simulink model "AUAV_V3_TestSensors"  (R2015a)
settings: Solver=FixedStepDiscrete  StartTime=0.0  StopTime=10.0  FixedStep=T  RelTol=1e-3
PreLoadFcn:
  | %T = 0.0025;
  | MavlinkBus;
  | mcuInit;
  | % Baro Altitude Computation
  | % =========================
  | basePressure = 98192.64;
  | baseTemp = 288.215;
  | lapseRate = -0.00198122;
  | baseHeight = 0;
values from neighbouring files (symbols this model uses):
  apSampleTime = 0.01    [mcuInit.m]
  latlong_WP = 1    [mcuInit.m]
  mavlink_attitude_t = Simulink.Bus    [MavlinkBusMarcello.m]
  mavlink_gps_raw_int_t = Simulink.Bus    [MavlinkBus.m]    (also in MavlinkBusMarcello.m)
  mavlink_raw_imu_t = Simulink.Bus    [MavlinkBus.m]    (also in MavlinkBusMarcello.m)
  mavlink_scaled_pressure_t = Simulink.Bus    [MavlinkBus.m]    (also in MavlinkBusMarcello.m)
  mavlink_servo_output_raw_t = Simulink.Bus    [MavlinkBusMarcello.m]
  mavlink_slugs_navigation_t = Simulink.Bus    [MavlinkBusMarcello.m]
  mavlink_sys_status_t = Simulink.Bus    [MavlinkBus.m]    (also in MavlinkBusMarcello.m)
  T = 0.01    [mcuInit.m]
  Xpoints = [0 0]    [mcuInit.m]
  Ypoints = [0 0]    [mcuInit.m]
  Zpoints = [0 0]    [mcuInit.m]
undefined symbols (not defined in the file or in its folder): A0, A14, A15, A2, A3, A4, A5, A6, accBiasRateLimit, B0, bankCommandLimit, barAdjust, baroCutoff, baroCutTemp, cubeAccelGain16405, cubeGyroGain16405, cubeMagGain16405, D0, D11, D7, D8, daLimit, data, daTrimMax, daTrimMin, deLimit, deTrimMax, deTrimMin, drLimit, drTrimMax, drTrimMin, dtLimit, dtTrimMax, dtTrimMin, F2, F3, G0, G13, G15, gaind, GS_location, gyroBiasRateLimit, IC1max, IPStar, ISA_g, Max, maxAcc, MaxDwnPthStar, maxDynPressure, maxEta, mlParamInterface, ms, OC1max, P112, P125, P127, P16, P20, P21, P30 ... (+26)
undefined symbols (not defined in the file): baroOffset, baroScale, barTGain1, barTGain2, barTMean1, barTMean2, bda, bde, bdr, bdt, bICda, bICde, bICdr, bICdt, derivativesConstant, lowRateSensorCutoff, mainSensorCutoff, mda, mde, mdr, mdt, mICda, mICde, mICdr, mICdt, pitotOffset, pitotScale, pitTGain1, pitTGain2, pitTMean1, pitTMean2, powerOffset, powerScale, pressureSensorCutoff, tempOffset, tempScale, vzCutoff, xCutoff, yCutoff
libraries: MCHP_Blockset x158, simulink x84, SLUGS_Library x31, aerolibconvert2 x6, aerolibutil x4, aerolibtransform2 x3, dspmtrx3 x2, aerolibobsolete x2
(part 2 of 24)

== system AUAV_V3_TestSensors/Barometer_Driver ==
  In1 : Inport
  BMP 180 Temperature Compensation See datasheet : Subsystem
  "BUS I2C Initialize BMP180 Read P, Convert T° @100Hz" : MCHP_Blockset/BUS I2C/BUS I2C MASTER  I2CRef=2  I2C_IntPriority=6  I2Csequence_txt="Initial-Configuration$     ---     $Start$Write Address:{[0x77]}    % BMP180 Address$Write Data (x1)  Write:{[0xF6]}  $Re-Start    % Re-Start when not followed with either Read or Write action rethrow Address$Read Data (x2)  Read:{adc out}    % Read converted value$Stop$Start$Write Address:{[0x77]}    % BMP180 Address$Write Data (x1)  Write:{[0xF4 0x2E]}      % Start T° Conversion$Stop"  I2Csequence_num=[BFF0000000000000 40E0600000000000 40F86A0000000000 410065D9C7810E65]$[4070000000000000]$[3FF0000000000000 40E0200000000000 40F86A0000000000 40F866E066594CA2]$[4040000000000000 0000000000000000 0000000000000000 405DC00000000000]$[4050000000000000 3FF0000000000000 0000000000000000 406EC00000000000]$[4008000000000000 40E0000000000000 40F86A0000000000 410065D9C7810E65]$[4060000000000000 4000000000000000]$[4000000000000000 40E0000000000000 40F86A0000000000 410065D9C7810E65]$[3FF0000000000000 40E0000000000000 40F86A0000000000 410065D9C7810E65]$[4040000000000000 0000000000000000 0000000000000000 405DC00000000000]$[4050000000000000 3FF0000000000000 0000000000000000 406E800000000000 4047000000000000]$[4000000000000000 40E0000000000000 40F86A0000000000 410065D9C7810E65]  InitialConfigurationNum=0  PIN_SDA_TXT=A3 / Pin[59]  PIN_SCL_TXT=A2 / Pin[58]  S_INPUT="[5  5]"  S_OUTPUT=[5]  S_INPUT_Size="[2  2]"  S_OUTPUT_Size=[4]  BlockingMode=off  SampleTime=[.01]  MCHP_MASTERLINK=|  MCHP_PORT={I2C 2 Clock}{SCL2}13:0:A2;{I2C 2 SDA}{SDA2}13:0:A3;  ORDERING=0
      | AUAV_V3_TestSensors/Microchip Master
      | AUAV V3 Board
      | Busy Flag on D2 (RA6)
  "BUS I2C Initialize BMP180 Read T°, Convert P @ 100Hz" : MCHP_Blockset/BUS I2C/BUS I2C MASTER  I2CRef=2  I2C_IntPriority=6  I2Csequence_txt="Initial-Configuration$     ---     $Start$Write Address:{[0x77]}    % BMP180 Address$Write Data (x1)  Write:{[0xF6]}  $Re-Start    % Re-Start when not followed with either Read or Write action rethrow Address$Read Data (x2)  Read:{adc out}    % Read converted value$Stop$Start$Write Address:{[0x77]}    % BMP180 Address$Write Data (x1)  Write:{[0xF4 0x34]}      % Start T° Conversion$Stop"  I2Csequence_num=[BFF0000000000000 40E0600000000000 40F86A0000000000 410065D9C7810E65]$[4070000000000000]$[3FF0000000000000 40E0200000000000 40F86A0000000000 40F866E066594CA2]$[4040000000000000 0000000000000000 0000000000000000 405DC00000000000]$[4050000000000000 3FF0000000000000 0000000000000000 406EC00000000000]$[4008000000000000 40E0000000000000 40F86A0000000000 410065D9C7810E65]$[4060000000000000 4000000000000000]$[4000000000000000 40E0000000000000 40F86A0000000000 410065D9C7810E65]$[3FF0000000000000 40E0000000000000 40F86A0000000000 410065D9C7810E65]$[4040000000000000 0000000000000000 0000000000000000 405DC00000000000]$[4050000000000000 3FF0000000000000 0000000000000000 406E800000000000 404A000000000000]$[4000000000000000 40E0000000000000 40F86A0000000000 410065D9C7810E65]  InitialConfigurationNum=0  PIN_SDA_TXT=A3 / Pin[59]  PIN_SCL_TXT=A2 / Pin[58]  S_INPUT="[5  5]"  S_OUTPUT=[5]  S_INPUT_Size="[2  2]"  S_OUTPUT_Size=[4]  BlockingMode=off  SampleTime=[.01]  MCHP_MASTERLINK=|  MCHP_PORT={I2C 2 Clock}{SCL2}13:0:A2;{I2C 2 SDA}{SDA2}13:0:A3;  ORDERING=0
      | AUAV_V3_TestSensors/Microchip Master
      | AUAV V3 Board
      | Busy Flag on D2 (RA6)
  Baro Altimeter : Subsystem  AncestorBlock=SLUGS_Library/Sensor Blocks/Baro Alt/Baro Altimeter
  Constant : Constant  Value=0  OutDataTypeStr=uint16
  Data Type Conversion10 : DataTypeConversion  OutDataTypeStr=int16
  Data Type Conversion7 : DataTypeConversion  OutDataTypeStr=int16
  Data Type Conversion8 : DataTypeConversion  OutDataTypeStr=int16
  Data Type Conversion9 : DataTypeConversion  OutDataTypeStr=single
  Delay : Delay  DelayLength=1  InitialCondition=1  InputProcessing=Inherited  SampleTime=.01
  Demux4 : Demux  Outputs=2
  Demux5 : Demux  Outputs=2
  Disable path through in HIL Subsystem : Subsystem  TreatAsAtomicUnit=on
  Disable path through in HIL Subsystem1 : Subsystem  TreatAsAtomicUnit=on
  Gain21 : Gain  Gain=10  OutDataTypeStr=int16
  I2C Initialisation Read EEPROM Calibration data Once (Blocking Function) : Subsystem
  LPF 1Hz : Subsystem  Tag=FilterWizardSubSystem
      settings: ErrorFcn=dspFilterRealizedInBasicElemsAlgLoopErrFcnCallback
  LPF 1Hz1 : Subsystem  Tag=FilterWizardSubSystem
      settings: ErrorFcn=dspFilterRealizedInBasicElemsAlgLoopErrFcnCallback
  Logical Operator : Logic  Operator=NOT  AllPortsSameDT=off  OutDataTypeStr=boolean
  Pack : Subsystem
  Pack1 : Subsystem
  Rate Transition1 : RateTransition  Deterministic=off  OutPortSampleTime=.01
  Script Pressure to Altitude : simulink/Model-Wide Utilities/DocBlock  DocumentType=Text
      content=|
      | %% The script to compute the lookup table to translate pressure from Pascal unit (Pa) to meters (m) here after
      |
      | func = '44331.5-4946.62*x.^0.190263';   % Model from Pressure (Pa) to altitude (m)
      |
      | xmin = 35000;  xmax = 101325; % Min and max pressure
      | xdt = ufix(32); xscale = 1; % x scaling
      |
      | ydt = ufix(16);
      | yscale = 2^-3;  % y output is altitude, in m. Max value is 8000 thus 13 bits are required for integer part and 3 can be used as fractional part.
      | % y LSB is 12.5 cm
      |
      | rndmeth = 'Floor';
      | errmax = [.2];
      | nptsmax = 256;
      | %spacing = 'even';
      |
      | % Compute lookup table (might take few seconds to compute)
      | [xdata,ydata,errworst] = fixpt_look1_func_approx(func,xmin,xmax,xdt,xscale,ydt,yscale,rndmeth,errmax,nptsmax);
      | % Check results
      | fixpt_look1_func_plot(xdata,ydata,func,xmin,xmax,xdt,xscale,ydt,yscale,rndmeth);
  wires:
  "BUS I2C Initialize BMP180 Read T°, Convert P @ 100Hz"/1 -> Demux4/1
  "BUS I2C Initialize BMP180 Read P, Convert T° @100Hz"/1 -> Demux5/1
  Demux4/1 -> Pack/1(Hi)
  Demux4/2 -> Pack/2(Low)
  Demux5/1 -> Pack1/1(Hi)
  Demux5/2 -> Pack1/2(Low)
  Pack1/1(Out1) -> LPF 1Hz1/1(Input)  "UP"
  Pack/1(Out1) -> LPF 1Hz/1(Input)  "UT"
  LPF 1Hz/1(Output) -> Data Type Conversion7/1, BMP 180 Temperature Compensation See datasheet/12(UT)  "U3 CH3"
  LPF 1Hz1/1(Output) -> Rate Transition1/1
  BMP 180 Temperature Compensation See datasheet/2(p) -> Baro Altimeter/1(Static (Pa))  "Pressute (Pa)"
  Constant/1 -> Delay/1
  I2C Initialisation Read EEPROM Calibration data Once (Blocking Function)/1(Out1) -> BMP 180 Temperature Compensation See datasheet/1(AC1)
  I2C Initialisation Read EEPROM Calibration data Once (Blocking Function)/2(Out2) -> BMP 180 Temperature Compensation See datasheet/2(AC2)
  I2C Initialisation Read EEPROM Calibration data Once (Blocking Function)/3(Out3) -> BMP 180 Temperature Compensation See datasheet/3(AC3)
  I2C Initialisation Read EEPROM Calibration data Once (Blocking Function)/4(Out4) -> BMP 180 Temperature Compensation See datasheet/4(AC4)
  I2C Initialisation Read EEPROM Calibration data Once (Blocking Function)/5(Out5) -> BMP 180 Temperature Compensation See datasheet/5(AC5)
  I2C Initialisation Read EEPROM Calibration data Once (Blocking Function)/6(Out6) -> BMP 180 Temperature Compensation See datasheet/6(AC6)
  I2C Initialisation Read EEPROM Calibration data Once (Blocking Function)/7(Out7) -> BMP 180 Temperature Compensation See datasheet/7(B1)
  I2C Initialisation Read EEPROM Calibration data Once (Blocking Function)/8(Out8) -> BMP 180 Temperature Compensation See datasheet/8(B2)
  I2C Initialisation Read EEPROM Calibration data Once (Blocking Function)/9(Out9) -> BMP 180 Temperature Compensation See datasheet/9(MB)
  I2C Initialisation Read EEPROM Calibration data Once (Blocking Function)/10(Out10) -> BMP 180 Temperature Compensation See datasheet/10(MC)
  I2C Initialisation Read EEPROM Calibration data Once (Blocking Function)/11(Out11) -> BMP 180 Temperature Compensation See datasheet/11(MD)
  Delay/1 -> I2C Initialisation Read EEPROM Calibration data Once (Blocking Function)/Enable
  Rate Transition1/1 -> Data Type Conversion8/1, BMP 180 Temperature Compensation See datasheet/13(UP)  "U3 CH4"
  Data Type Conversion7/1 -> Disable path through in HIL Subsystem/1(In1)
  Data Type Conversion8/1 -> Disable path through in HIL Subsystem/2(In2)
  BMP 180 Temperature Compensation See datasheet/1(T) -> Gain21/1  "Temp (deg) * 10"
  Baro Altimeter/1(Altitude) -> Data Type Conversion9/1  "U3 CH3"
  Data Type Conversion10/1 -> Disable path through in HIL Subsystem1/1(In1)
  Gain21/1 -> Data Type Conversion10/1
  [HIL_FLAG] -> Logical Operator/1
  Logical Operator/1 -> Disable path through in HIL Subsystem1/Enable, Disable path through in HIL Subsystem/Enable
  Data Type Conversion9/1 -> Disable path through in HIL Subsystem1/2(In2)
  In1/1 -> [HIL_FLAG]

== system AUAV_V3_TestSensors/Control Surface Input ==
  Input Capture : MCHP_Blockset/Pulse Input//Output/Input Capture  IntPriority=6  Channel="[1     2     3     4     5]"  Channel_OLD="[1  2  3  4  5]"  PIN_IC1=Dynamic Options  PIN_IC1_TXT=D0 / P64 / Pin[72]  PIN_IC2=Dynamic Options  PIN_IC2_TXT=D8 / P72 / Pin[68]  PIN_IC3=Dynamic Options  PIN_IC3_TXT=D11 / P75 / Pin[71]  PIN_IC4=Dynamic Options  PIN_IC4_TXT=A15 / P31 / Pin[67]  PIN_IC5=Dynamic Options  PIN_IC5_TXT=A0 / P16 / Pin[17]  PIN_IC6=Dynamic Options  PIN_IC6_TXT=A0 / P16 / Pin[17]  PIN_IC7=Dynamic Options  PIN_IC7_TXT=A0 / P16 / Pin[17]  PIN_IC8=Dynamic Options  PIN_IC8_TXT=A0 / P16 / Pin[17]  PIN_IC9=Dynamic Options  PIN_IC9_TXT=A0 / P16 / Pin[17]  PIN_IC10=Dynamic Options  PIN_IC10_TXT=A0 / P16 / Pin[17]  PIN_IC11=Dynamic Options  PIN_IC11_TXT=A0 / P16 / Pin[17]  PIN_IC12=Dynamic Options  PIN_IC12_TXT=A0 / P16 / Pin[17]  PIN_IC13=Dynamic Options  PIN_IC13_TXT=A0 / P16 / Pin[17]  PIN_IC14=Dynamic Options  PIN_IC14_TXT=A0 / P16 / Pin[17]  PIN_IC15=Dynamic Options  PIN_IC15_TXT=A0 / P16 / Pin[17]  PIN_IC16=Dynamic Options  PIN_IC16_TXT=A0 / P16 / Pin[17]  Channel_UP_Down_Periode="[1     1     1     1     1]"  MaxChannel="[0.003   0.003   0.003   0.003   0.003]"  SafeMarge="[0     0     0     0     0]"  MaxChannelValue="2.^[ 14.680  14.680  14.680  14.680  14.680]  =>  [26249  26249  26249  26249  26249]"  ICxmax="[26249  26249  26249  26249  26249]"  Timer="[1  1  1  1  1]"  ChangeDetected="[0     0     0     0     0]"  ChangeDetectedPortRef=3  SampleTime=.02  Status=OK  MCHP_PORT={Input Capture 1}{IC1}6:0:P64;{Input Capture 2}{IC2}6:0:P72;{Input Capture 3}{IC3}6:0:P75;{Input Capture 4}{IC4}6:0:P31;{Input Capture 5}{IC5}6:0:P16;  MCHP_TIMER_REQUEST="{Input Capture 1}{IC1}6:0:1:0:[1  2  3  4  5]:210000;{Input Capture 1}{IC1}6:0:1:0:[1  2  3  4  5]:210000;{Input Capture 1}{IC1}6:0:1:0:[1  2  3  4  5]:210000;{Input Capture 1}{IC1}6:0:1:0:[1  2  3  4  5]:210000;{Input Capture 1}{IC1}6:0:1:0:[1  2  3  4  5]:210000;"  MCHP_TIMER_RESULT=[1 26249.000000000011 ;1 26249.000000000011 ;1 26249.000000000011 ;1 26249.000000000011 ;1 26249.000000000011 ]  MCHP_MASTERLINK=|
      | AUAV_V3_TestSensors/Microchip Master
      | AUAV V3 Board
      | Busy Flag on D2 (RA6)
  PilotConsole : Subsystem  TreatAsAtomicUnit=on
      settings: RTWFileNameOpts=Use subsystem name
  Pilot Console : Outport
  wires:
  Input Capture/1 -> PilotConsole/1(In1)  "dT"
  Input Capture/2 -> PilotConsole/2(In2)  "dA"
  Input Capture/3 -> PilotConsole/3(In3)  "dE"
  Input Capture/4 -> PilotConsole/4(In4)  "dR"
  Input Capture/5 -> PilotConsole/5(In5)  "dFailsafe"
  PilotConsole/1(Pilot Console) -> Pilot Console/1

== system AUAV_V3_TestSensors/IMU_Mag_Driver ==
  In1 : Inport
  BUS I2C Read HMC5883 Magn (100 Hz)1 : MCHP_Blockset/BUS I2C/BUS I2C MASTER  I2CRef=2  I2C_IntPriority=6  I2Csequence_txt="Initial-Configuration$     ---     $Start$Write Address:{[0x1E]}    % HMC5883L Address$Write Data (x1)  Write:{[0x3]}  $Stop$Start$Write Address:{[0x1E]}    % HMC5883L Address$Read Data (x6)  Read:{Out 5}$Stop"  I2Csequence_num=[BFF0000000000000 40E0600000000000 40F86A0000000000 410065D9C7810E65]$[4070000000000000]$[3FF0000000000000 40E0200000000000 40F86A0000000000 40F866E066594CA2]$[4040000000000000 0000000000000000 0000000000000000 403E000000000000]$[4050000000000000 3FF0000000000000 0000000000000000 4008000000000000]$[4000000000000000 40E0600000000000 40F86A0000000000 40F866E066594CA2]$[3FF0000000000000 40E0200000000000 40F86A0000000000 40F866E066594CA2]$[4040000000000000 0000000000000000 0000000000000000 403E000000000000]$[4060000000000000 4018000000000000]$[4000000000000000 40E0600000000000 40F86A0000000000 40F866E066594CA2]  InitialConfigurationNum=0  PIN_SDA_TXT=A3 / Pin[59]  PIN_SCL_TXT=A2 / Pin[58]  S_INPUT="[5  5]"  S_OUTPUT=[5]  S_INPUT_Size="[2  2]"  S_OUTPUT_Size=[4]  BlockingMode=off  SampleTime=[.01]  MCHP_MASTERLINK=|  MCHP_PORT={I2C 2 Clock}{SCL2}13:0:A2;{I2C 2 SDA}{SDA2}13:0:A3;  ORDERING=0
      | AUAV_V3_TestSensors/Microchip Master
      | AUAV V3 Board
      | Busy Flag on D2 (RA6)
  BUS I2C Read HMC5883 Magn (50 Hz) : MCHP_Blockset/BUS I2C/BUS I2C MASTER  Commented=on  I2CRef=2  I2C_IntPriority=6  I2Csequence_txt="Initial-Configuration$     ---     $Start$Write Address:{[0x1E]}    % HMC5883L Address$Write Data (x1)  Write:{[0x3]}  $Stop$Start$Write Address:{[0x1E]}    % HMC5883L Address$Read Data (x6)  Read:{Out 5}$Stop"  I2Csequence_num=[BFF0000000000000 40E0600000000000 41186A0000000000 4118666E3C87173F]$[4070000000000000]$[3FF0000000000000 40E0200000000000 40F86A0000000000 40F866E066594CA2]$[4040000000000000 0000000000000000 0000000000000000 403E000000000000]$[4050000000000000 3FF0000000000000 0000000000000000 4008000000000000]$[4000000000000000 40E0600000000000 40F86A0000000000 40F866E066594CA2]$[3FF0000000000000 40E0200000000000 40F86A0000000000 40F866E066594CA2]$[4040000000000000 0000000000000000 0000000000000000 403E000000000000]$[4060000000000000 4018000000000000]$[4000000000000000 40E0600000000000 40F86A0000000000 40F866E066594CA2]  InitialConfigurationNum=0  PIN_SDA_TXT=A3 / Pin[59]  PIN_SCL_TXT=A2 / Pin[58]  S_INPUT="[5  5]"  S_OUTPUT=[5]  S_INPUT_Size="[2  2]"  S_OUTPUT_Size=[4]  BlockingMode=off  SampleTime=0.01  MCHP_MASTERLINK=|  MCHP_PORT={I2C 2 Clock}{SCL2}13:0:A2;{I2C 2 SDA}{SDA2}13:0:A3;  ORDERING=0
      | AUAV_V3_TestSensors/Microchip Master
      | AUAV V3 Board
      | Busy Flag on D2 (RA6)
  "BUS SPI Read MPU 6050 Axyz, T°, Gxyz (1 kHz)" : MCHP_Blockset/BUS SPI/BUS SPI  Commented=on  SPIRef=1  DMA="[0  2  3]"  SPI_IntPriority=5  SPIsequence_txt="Initial-Configuration$     ---     $Set Port E4 / Pin[100] to 0    % /CS$Write only (x1)  Write:{[0xBA00]}      % read one byte before$Read only (x3)  Read:{Axyz}    % Accelerometers$Read only (x1)  Read:{T°}    % Temperature$Read only (x3)  Read:{Gxyz}    % rate gyros$Set Port E4 / Pin[100] to 1    % /CS"  SPIsequence_num=[BFF0000000000000 4091D00000000000 0000000000000000 40E0000000000000 4116409C00000000 4116409D55555555]$[4070000000000000]$[4010000000000000 4051000000000000 0000000000000000]$[3FF0000000000000 3FF0000000000000 0000000000000000 40E7400000000000]$[4000000000000000 4008000000000000]$[4000000000000000 3FF0000000000000]$[4000000000000000 4008000000000000]$[4010000000000000 4051000000000000 3FF0000000000000]  PIN_SDI_TXT=E3 / P83 / Pin[99]  PIN_SDO_TXT=E2 / P82 / Pin[98]  PIN_SCK_TXT=G15 / P127 / Pin[1]  PIN_SS_TXT=B0 / Pin[21]  S_INPUT="[5  5]"  S_OUTPUT=[5]  S_INPUT_Size="[2  2]"  S_OUTPUT_Size=[4]  BlockingMode=off  SampleTime=[.01]  MCHP_MASTERLINK=|  MCHP_PORT={SPI 1 input}{SDI1}12:0:P83;{SPI 1 output}{SDO1}12:1:P82;{SPI 1 Clock output}{SCK1}12:1:P127;{SPI 1 Digital output}{SPI1-DOU}12:1:E4;{SPI 1 Digital output}{SPI1-DOU}12:1:E4;  ORDERING=0
      | AUAV_V3_TestSensors/Microchip Master
      | AUAV V3 Board
      | Busy Flag on D2 (RA6)
  BUS SPI Read MPU 6050 : Subsystem
  Data Type Conversion{,1..5} (6 alike) : DataTypeConversion  Commented=on  OutDataTypeStr=int16
  Data Type Conversion{6..11} (6 alike) : DataTypeConversion  OutDataTypeStr=int16
  Demux1 : Demux  Commented=on  Outputs=3
  Demux2 : Demux  Commented=on  Outputs=3
  Demux3 : Demux  Commented=on  Outputs=6
  Demux4 : Demux  Outputs=3
  Demux5 : Demux  Outputs=3
  Demux6 : Demux  Outputs=6
  Disable path through in HIL Subsystem1 : Subsystem  TreatAsAtomicUnit=on
  Logical Operator1 : Logic  Operator=NOT  AllPortsSameDT=off  OutDataTypeStr=boolean
  Rate Transition : RateTransition
  Subsystem1 : Subsystem
  Subsystem10 : Subsystem  Commented=on
  Subsystem2 : Subsystem
  Subsystem3 : Subsystem
  Subsystem8 : Subsystem  Commented=on
  Subsystem9 : Subsystem  Commented=on
  Update MPU_T : DataStoreWrite  Commented=on  DataStoreName=MPU_T  DataStoreElements=MPU_T
  Update Raw IMU DATA : DataStoreWrite  Commented=on  DialogController=Simulink.DDGSource  DataStoreName=mlRawImuData  DataStoreElements=mlRawIMU.xacc#mlRawIMU.yacc#mlRawIMU.zacc#mlRawIMU.xgyro#mlRawIMU.ygyro#mlRawIMU.zgyro#mlRawIMU.xmag#mlRawIMU.ymag#mlRawIMU.zmag
  wires:
  "BUS SPI Read MPU 6050 Axyz, T°, Gxyz (1 kHz)"/1 -> Demux1/1  "U1 CH8"
  "BUS SPI Read MPU 6050 Axyz, T°, Gxyz (1 kHz)"/3 -> Demux2/1
  Demux1/3 -> Data Type Conversion2/1  "U1 CH3"
  Demux1/1 -> Data Type Conversion/1  "U1 CH1"
  Demux1/2 -> Data Type Conversion1/1  "U1 CH2"
  Demux2/1 -> Data Type Conversion3/1  "U1 CH5"
  Demux2/2 -> Data Type Conversion4/1  "U1 CH6"
  Demux2/3 -> Data Type Conversion5/1  "U1 CH7"
  BUS I2C Read HMC5883 Magn (50 Hz)/1 -> Demux3/1
  Demux3/1 -> Subsystem8/1(Hi)
  Demux3/2 -> Subsystem8/2(Low)
  Demux3/3 -> Subsystem9/1(Hi)
  Demux3/4 -> Subsystem9/2(Low)
  Demux3/6 -> Subsystem10/2(Low)
  Demux3/5 -> Subsystem10/1(Hi)
  Subsystem9/1(Out1) -> Update Raw IMU DATA/8  "U1 CH9"
  Subsystem8/1(Out1) -> Update Raw IMU DATA/7  "U1 CH8"
  Subsystem10/1(Out1) -> Update Raw IMU DATA/9  "U1 CH10"
  Data Type Conversion/1 -> Update Raw IMU DATA/1
  Data Type Conversion1/1 -> Update Raw IMU DATA/2
  Data Type Conversion2/1 -> Update Raw IMU DATA/3
  Data Type Conversion3/1 -> Update Raw IMU DATA/4
  Data Type Conversion4/1 -> Update Raw IMU DATA/5
  Data Type Conversion5/1 -> Update Raw IMU DATA/6
  "BUS SPI Read MPU 6050 Axyz, T°, Gxyz (1 kHz)"/2 -> Update MPU_T/1  "U1 CH4"
  Demux6/1 -> Subsystem2/1(Hi)
  Demux6/2 -> Subsystem2/2(Low)
  Demux6/3 -> Subsystem3/1(Hi)
  Demux6/4 -> Subsystem3/2(Low)
  Demux6/6 -> Subsystem1/2(Low)
  Demux6/5 -> Subsystem1/1(Hi)
  BUS SPI Read MPU 6050/4(Axyz RAW) -> Demux4/1
  Demux4/3 -> Data Type Conversion8/1  "U1 CH3"
  Demux4/1 -> Data Type Conversion6/1  "U1 CH1"
  Demux4/2 -> Data Type Conversion7/1  "U1 CH2"
  Demux5/1 -> Data Type Conversion9/1  "U1 CH5"
  Demux5/2 -> Data Type Conversion10/1  "U1 CH6"
  Demux5/3 -> Data Type Conversion11/1  "U1 CH7"
  Subsystem3/1(Out1) -> Disable path through in HIL Subsystem1/8(In8)  "U1 CH9"
  Subsystem2/1(Out1) -> Disable path through in HIL Subsystem1/7(In7)  "U1 CH8"
  Subsystem1/1(Out1) -> Disable path through in HIL Subsystem1/9(In9)  "U1 CH10"
  Data Type Conversion6/1 -> Disable path through in HIL Subsystem1/1(In1)
  Data Type Conversion7/1 -> Disable path through in HIL Subsystem1/2(In2)
  Data Type Conversion8/1 -> Disable path through in HIL Subsystem1/3(In3)
  Data Type Conversion9/1 -> Disable path through in HIL Subsystem1/4(In4)
  Data Type Conversion10/1 -> Disable path through in HIL Subsystem1/5(In5)
  Data Type Conversion11/1 -> Disable path through in HIL Subsystem1/6(In6)
  Rate Transition/1 -> Demux6/1
  BUS SPI Read MPU 6050/3(T) -> Disable path through in HIL Subsystem1/10(In10)
  BUS I2C Read HMC5883 Magn (100 Hz)1/1 -> Rate Transition/1
  In1/1 -> [HIL_FLAG]
  [HIL_FLAG] -> Logical Operator1/1
  Logical Operator1/1 -> Disable path through in HIL Subsystem1/Enable
  BUS SPI Read MPU 6050/5(Gxyz RAW) -> Demux5/1

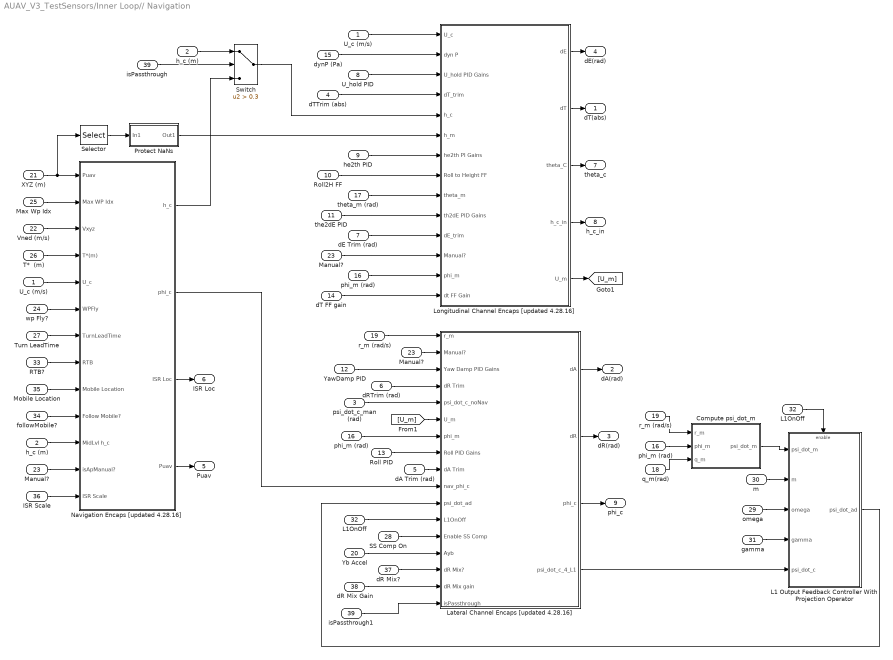
== system AUAV_V3_TestSensors/Inner Loop// Navigation ==
  U_c (m/s) : Inport
  h_c (m) : Inport  Port=2
  psi_dot_c_man (rad) : Inport  Port=3
  dTTrim (abs) : Inport  Port=4
  dA Trim (rad) : Inport  Port=5
  dRTrim (rad) : Inport  Port=6
  dE Trim (rad) : Inport  Port=7
  U_hold PID : Inport  Port=8
  he2th PID : Inport  Port=9
  Roll2H FF : Inport  Port=10
  the2dE PID : Inport  Port=11
  YawDamp PID : Inport  Port=12
  "Roll PID " : Inport  Port=13
  dT FF gain : Inport  Port=14
  dynP (Pa) : Inport  Port=15
  phi_m (rad) : Inport  Port=16
  theta_m (rad) : Inport  Port=17
  q_m(rad) : Inport  Port=18
  r_m (rad/s) : Inport  Port=19
  Yb Accel : Inport  Port=20
  XYZ (m) : Inport  Port=21
  Vned (m/s) : Inport  Port=22
  Manual? : Inport  Port=23
  wp Fly? : Inport  Port=24
  Max Wp Idx : Inport  Port=25
  T*  (m) : Inport  Port=26
  Turn LeadTime : Inport  Port=27
  SS Comp On : Inport  Port=28
  omega : Inport  Port=29
  m : Inport  Port=30
  gamma : Inport  Port=31
  L1OnOff : Inport  Port=32
  RTB? : Inport  Port=33
  followMobile? : Inport  Port=34
  Mobile Location : Inport  Port=35
  ISR Scale : Inport  Port=36
  dR Mix? : Inport  Port=37
  dR Mix Gain : Inport  Port=38
  isPassthrough : Inport  Port=39
  Compute psi_dot_m : Subsystem
  L1 Output Feedback Controller With Projection Operator : Subsystem  TreatAsAtomicUnit=on
  "L1OnOff " : InportShadow  Port=32
  Lateral Channel Encaps [updated 4.28.16] : Subsystem  TreatAsAtomicUnit=on
  Longitudinal Channel Encaps [updated 4.28.16] : Subsystem  TreatAsAtomicUnit=on
  "Manual? " : InportShadow  Port=23
  "Manual?  " : InportShadow  Port=23
  Navigation Encaps [updated 4.28.16] : Subsystem  TreatAsAtomicUnit=on
  Protect NaNs : Subsystem
  Selector : Selector  InputPortWidth=3  Indices=[3]
  Switch : Switch  Criteria=u2 > Threshold  Threshold=0.3  OutDataTypeStr=Inherit: Inherit via back propagation  InputSameDT=on
  "U_c (m/s) " : InportShadow
  "h_c (m) " : InportShadow  Port=2
  isPassthrough1 : InportShadow  Port=39
  "phi_m (rad) " : InportShadow  Port=16
  "phi_m (rad)   " : InportShadow  Port=16
  "r_m (rad/s) " : InportShadow  Port=19
  dT(abs) : Outport
  dA(rad) : Outport  Port=2
  dR(rad) : Outport  Port=3
  dE(rad) : Outport  Port=4
  "Puav " : Outport  Port=5
  ISR Loc : Outport  Port=6
  theta_c : Outport  Port=7
  h_c_in : Outport  Port=8
  phi_c : Outport  Port=9
  wires:
  Manual?/1 -> Longitudinal Channel Encaps [updated 4.28.16]/12(Manual?)
  U_c (m/s)/1 -> Longitudinal Channel Encaps [updated 4.28.16]/1(U_c)
  dynP (Pa)/1 -> Longitudinal Channel Encaps [updated 4.28.16]/2(dyn P)
  Longitudinal Channel Encaps [updated 4.28.16]/1(dE) -> dE(rad)/1
  U_hold PID/1 -> Longitudinal Channel Encaps [updated 4.28.16]/3(U_hold PID Gains)
  dTTrim (abs)/1 -> Longitudinal Channel Encaps [updated 4.28.16]/4(dT_trim)
  Longitudinal Channel Encaps [updated 4.28.16]/2(dT) -> dT(abs)/1
  Selector/1 -> Protect NaNs/1(In1)
  he2th PID/1 -> Longitudinal Channel Encaps [updated 4.28.16]/7(he2th PI Gains)
  theta_m (rad)/1 -> Longitudinal Channel Encaps [updated 4.28.16]/9(theta_m)
  Longitudinal Channel Encaps [updated 4.28.16]/3(theta_C) -> theta_c/1
  the2dE PID/1 -> Longitudinal Channel Encaps [updated 4.28.16]/10(th2dE PID Gains)
  dE Trim (rad)/1 -> Longitudinal Channel Encaps [updated 4.28.16]/11(dE_trim)
  Longitudinal Channel Encaps [updated 4.28.16]/4(h_c_in) -> h_c_in/1
  r_m (rad/s)/1 -> Lateral Channel Encaps [updated 4.28.16]/1(r_m)
  YawDamp PID/1 -> Lateral Channel Encaps [updated 4.28.16]/3(Yaw Damp PID Gains)
  dRTrim (rad)/1 -> Lateral Channel Encaps [updated 4.28.16]/4(dR Trim)
  Lateral Channel Encaps [updated 4.28.16]/2(dR) -> dR(rad)/1
  psi_dot_c_man (rad)/1 -> Lateral Channel Encaps [updated 4.28.16]/5(psi_dot_c_noNav)
  phi_m (rad)/1 -> Lateral Channel Encaps [updated 4.28.16]/7(phi_m)
  Lateral Channel Encaps [updated 4.28.16]/3(phi_c) -> phi_c/1
  "Roll PID "/1 -> Lateral Channel Encaps [updated 4.28.16]/8(Roll PID Gains)
  dA Trim (rad)/1 -> Lateral Channel Encaps [updated 4.28.16]/9(dA Trim)
  Longitudinal Channel Encaps [updated 4.28.16]/5(U_m) -> [U_m]
  XYZ (m)/1 -> Selector/1, Navigation Encaps [updated 4.28.16]/1(Puav)
  Max Wp Idx/1 -> Navigation Encaps [updated 4.28.16]/2(Max WP Idx)
  Vned (m/s)/1 -> Navigation Encaps [updated 4.28.16]/3(Vxyz)
  Compute psi_dot_m/1(psi_dot_m) -> L1 Output Feedback Controller With Projection Operator/1(psi_dot_m)
  m/1 -> L1 Output Feedback Controller With Projection Operator/2(m)
  omega/1 -> L1 Output Feedback Controller With Projection Operator/3(omega)
  gamma/1 -> L1 Output Feedback Controller With Projection Operator/4(gamma)
  "r_m (rad/s) "/1 -> Compute psi_dot_m/1(r_m)
  "phi_m (rad) "/1 -> Compute psi_dot_m/2(phi_m)
  q_m(rad)/1 -> Compute psi_dot_m/3(q_m)
  L1OnOff/1 -> L1 Output Feedback Controller With Projection Operator/Enable
  L1 Output Feedback Controller With Projection Operator/1(psi_dot_ad) -> Lateral Channel Encaps [updated 4.28.16]/11(psi_dot_ad)
  "L1OnOff "/1 -> Lateral Channel Encaps [updated 4.28.16]/12(L1OnOff)
  "phi_m (rad)   "/1 -> Longitudinal Channel Encaps [updated 4.28.16]/13(phi_m)
  dT FF gain/1 -> Longitudinal Channel Encaps [updated 4.28.16]/14(dt FF Gain)
  Lateral Channel Encaps [updated 4.28.16]/1(dA) -> dA(rad)/1
  SS Comp On/1 -> Lateral Channel Encaps [updated 4.28.16]/13(Enable SS Comp)
  Yb Accel/1 -> Lateral Channel Encaps [updated 4.28.16]/14(Ayb)
  Lateral Channel Encaps [updated 4.28.16]/4(psi_dot_c_4_L1) -> L1 Output Feedback Controller With Projection Operator/5(psi_dot_c)
  Protect NaNs/1(Out1) -> Longitudinal Channel Encaps [updated 4.28.16]/6(h_m)
  [U_m] -> Lateral Channel Encaps [updated 4.28.16]/6(U_m)
  "Manual?  "/1 -> Lateral Channel Encaps [updated 4.28.16]/2(Manual?)
  Roll2H FF/1 -> Longitudinal Channel Encaps [updated 4.28.16]/8(Roll to Height FF)
  Navigation Encaps [updated 4.28.16]/2(phi_c) -> Lateral Channel Encaps [updated 4.28.16]/10(nav_phi_c)
  T*  (m)/1 -> Navigation Encaps [updated 4.28.16]/4(T*(m))
  "U_c (m/s) "/1 -> Navigation Encaps [updated 4.28.16]/5(U_c)
  wp Fly?/1 -> Navigation Encaps [updated 4.28.16]/6(WPFly)
  Turn LeadTime/1 -> Navigation Encaps [updated 4.28.16]/7(TurnLeadTime)
  RTB?/1 -> Navigation Encaps [updated 4.28.16]/8(RTB)
  Mobile Location/1 -> Navigation Encaps [updated 4.28.16]/9(Mobile Location)
  followMobile?/1 -> Navigation Encaps [updated 4.28.16]/10(Follow Mobile?)
  "h_c (m) "/1 -> Navigation Encaps [updated 4.28.16]/11(MidLvl h_c)
  "Manual? "/1 -> Navigation Encaps [updated 4.28.16]/12(isApManual?)
  Navigation Encaps [updated 4.28.16]/3(ISR Loc) -> ISR Loc/1
  Navigation Encaps [updated 4.28.16]/4("Puav ") -> "Puav "/1
  dR Mix Gain/1 -> Lateral Channel Encaps [updated 4.28.16]/16(dR Mix gain)
  dR Mix?/1 -> Lateral Channel Encaps [updated 4.28.16]/15(dR Mix?)
  ISR Scale/1 -> Navigation Encaps [updated 4.28.16]/13(ISR Scale)
  isPassthrough/1 -> Switch/2
  h_c (m)/1 -> Switch/1
  Switch/1 -> Longitudinal Channel Encaps [updated 4.28.16]/5(h_c)
  Navigation Encaps [updated 4.28.16]/1(h_c) -> Switch/3
  isPassthrough1/1 -> Lateral Channel Encaps [updated 4.28.16]/17(isPassthrough)

== system AUAV_V3_TestSensors/LEDs_Driver ==
  LED 1 (Blue) : MCHP_Blockset/Digital IO/Digital Output  PORT=Dynamic Options  PORT_TXT="B   [ 0 : 15 ]"  PIN=2  PACK=off  SIMULTANEOUS=off  READPREVIOUS=on  ORDERING=None  SampleTime=.05  MCHP_MASTERLINK=|
      | AUAV_V3_TestSensors/Microchip Master
      | AUAV V3 Board
      | Busy Flag on D2 (RA6)
  LED 2 (red) : MCHP_Blockset/Digital IO/Digital Output  PORT=Dynamic Options  PORT_TXT="B   [ 0 : 15 ]"  PIN=3  PACK=off  SIMULTANEOUS=off  READPREVIOUS=on  ORDERING=None  SampleTime=.1  MCHP_MASTERLINK=|
      | AUAV_V3_TestSensors/Microchip Master
      | AUAV V3 Board
      | Busy Flag on D2 (RA6)
  LED 3 (Green) : MCHP_Blockset/Digital IO/Digital Output  PORT=Dynamic Options  PORT_TXT="B   [ 0 : 15 ]"  PIN=4  PACK=off  SIMULTANEOUS=off  READPREVIOUS=on  ORDERING=None  SampleTime=.25  MCHP_MASTERLINK=|
      | AUAV_V3_TestSensors/Microchip Master
      | AUAV V3 Board
      | Busy Flag on D2 (RA6)
  LED 4 (Yellow) : MCHP_Blockset/Digital IO/Digital Output  PORT=Dynamic Options  PORT_TXT="B   [ 0 : 15 ]"  PIN=5  PACK=off  SIMULTANEOUS=off  READPREVIOUS=on  ORDERING=None  SampleTime=0.5  MCHP_MASTERLINK=|
      | AUAV_V3_TestSensors/Microchip Master
      | AUAV V3 Board
      | Busy Flag on D2 (RA6)
  Logical Operator{,1..3} (4 alike) : Logic  Operator=NOT  AllPortsSameDT=off  OutDataTypeStr=boolean
  wires:
  LED 1 (Blue)/1 -> Logical Operator/1
  Logical Operator/1 -> LED 1 (Blue)/1
  LED 2 (red)/1 -> Logical Operator1/1
  Logical Operator1/1 -> LED 2 (red)/1
  LED 3 (Green)/1 -> Logical Operator2/1
  Logical Operator2/1 -> LED 3 (Green)/1
  LED 4 (Yellow)/1 -> Logical Operator3/1
  Logical Operator3/1 -> LED 4 (Yellow)/1
